simulink model "cv_5d_simulink_VA1"  (R2018a)
settings: Solver=VariableStepAuto  StartTime=0.0  StopTime=10  RelTol=1e-3
values from neighbouring files (symbols this model uses):
  b = 0.2    [cv_5a2_VA1.m]    (also in cv_5b_VA1.m; cv_5d_VA1.m = 10)
  k = 100    [cv_5a1_VA1.m]    (also in cv_5a2_VA1.m = 1; cv_5b_VA1.m = 1; cv_5d_VA1.m = 20)
  m = 100    [cv_5a1_VA1.m]    (also in cv_5a2_VA1.m = 1; cv_5b_VA1.m = 1; cv_5d_VA1.m = 1)
libraries: simulink x1
settings Model: Creator=Roman  LastModifiedBy=Roman

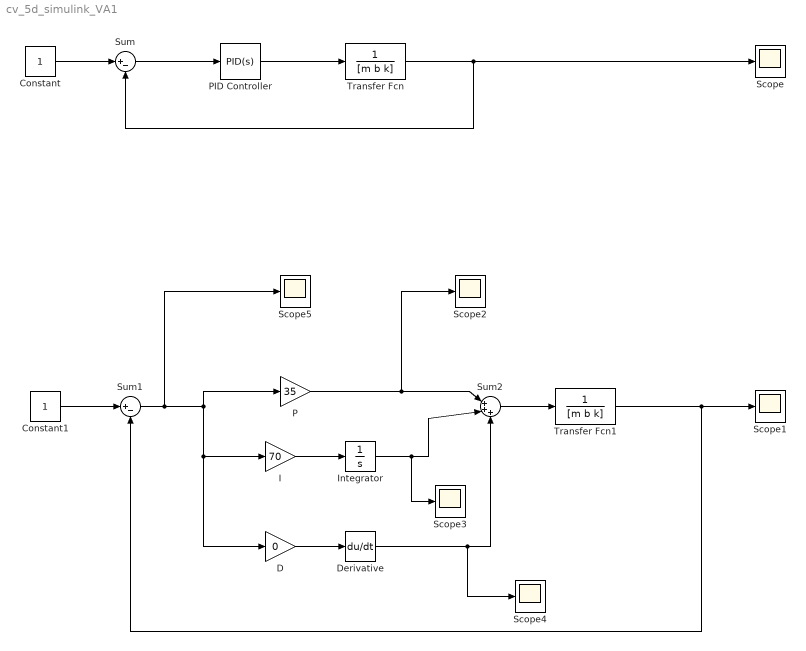
== system cv_5d_simulink_VA1 ==
  Constant : Constant
  Constant1 : Constant
  D : Gain  Gain=0
  Derivative : Derivative
  I : Gain  Gain=70
  Integrator : Integrator
  P : Gain  Gain=35
  PID Controller : simulink/Continuous/PID Controller  Controller=PID  TimeDomain=Continuous-time  SampleTime=-1  IntegratorMethod=Forward Euler  FilterMethod=Forward Euler  Form=Parallel  UseFilter=on  ControllerParametersSource=internal  P=30  I=70  D=0  N=100  InitialConditionSource=internal  InitialConditionForIntegrator=0  InitialConditionForFilter=0  ExternalReset=none  LimitOutput=off  UpperSaturationLimit=inf  LowerSaturationLimit=-inf  LinearizeAsGain=on  AntiWindupMode=none  Kb=1  TrackingMode=off  Kt=1  PParamMin=[]  PParamMax=[]  IParamMin=[]  IParamMax=[]  DParamMin=[]  DParamMax=[]  NParamMin=[]  NParamMax=[]  KbParamMin=[]  KbParamMax=[]  KtParamMin=[]  KtParamMax=[]  POutMin=[]  POutMax=[]  IOutMin=[]  IOutMax=[]  DOutMin=[]  DOutMax=[]  NOutMin=[]  NOutMax=[]  KbOutMin=[]  KbOutMax=[]  KtOutMin=[]  KtOutMax=[]  IntegratorOutMin=[]  IntegratorOutMax=[]  FilterOutMin=[]  FilterOutMax=[]  SumOutMin=[]  SumOutMax=[]  SumI1OutMin=[]  SumI1OutMax=[]  SumI2OutMin=[]  SumI2OutMax=[]  SumI3OutMin=[]  SumI3OutMax=[]  SumDOutMin=[]  SumDOutMax=[]  SaturationOutMin=[]  SaturationOutMax=[]  IntegratorContinuousStateAttributes=''  IntegratorStateMustResolveToSignalObject=off  IntegratorRTWStateStorageClass=Auto  FilterContinuousStateAttributes=''  FilterStateMustResolveToSignalObject=off  FilterRTWStateStorageClass=Auto  DifferentiatorICPrevScaledInput=0  DifferentiatorOutMin=[]  DifferentiatorOutMax=[]  FilterDiffOutCoefMin=[]  FilterDiffOutCoefMax=[]  SumDenOutMin=[]  SumDenOutMax=[]  SumNumOutMin=[]  SumNumOutMax=[]  ReciprocalOutMin=[]  ReciprocalOutMax=[]  DivideOutMin=[]  DivideOutMax=[]  TunerSelectOption=Transfer Function Based (PID Tuner App)
  Scope{,1..5} (6 alike) : Scope
  Sum : Sum  Inputs=|+-
  Sum1 : Sum  Inputs=|+-
  Sum2 : Sum  Inputs=|+++
  Transfer Fcn : TransferFcn  Denominator=[m b k]
  Transfer Fcn1 : TransferFcn  Denominator=[m b k]
  wires:
  Constant/1 -> Sum/1
  Sum/1 -> PID Controller/1
  PID Controller/1 -> Transfer Fcn/1
  Transfer Fcn/1 -> Sum/2, Scope/1
  Constant1/1 -> Sum1/1
  Transfer Fcn1/1 -> Sum1/2, Scope1/1
  Sum2/1 -> Transfer Fcn1/1
  P/1 -> Scope2/1, Sum2/1
  Sum1/1 -> Scope5/1, D/1, I/1, P/1
  I/1 -> Integrator/1
  Integrator/1 -> Scope3/1, Sum2/2
  D/1 -> Derivative/1
  Derivative/1 -> Scope4/1, Sum2/3
